simulink model "ALFlight3Wing"  (R2019a)
settings: Solver=VariableStepAuto  StartTime=0.0  StopTime=100  RelTol=1e-3
InitFcn:
  | Ts=.05
  | load('goodMPC.mat')
  | %load('fault2mpc.mat')
  | global counts
  | counts=0
  | 
  | An=[-0.0220400000000000,0.00142200000000000,0,-32.1700000000000,0,0,0,0,0,0;-0.0575900000000000,-0.394300000000000,871,0,0,0,0,0,0,0;-9.50000000000000e-05,-0.00179300000000000,-0.546800000000000,0,0,0,0,0,0,0;0,0,1,0,0,0,0,0,0,0;0,0,0,0,-0.0639900000000000,0,-1,0.0369100000000000,0,0;0,0,0,0,-2.11100000000000,-0.504800000000000,0.193000000000000,0,0,0;0,0,0,0,0.773200000000000,0.0108700000000000,-0.179400000000000,0,0,0;0,0,0,0,0,1,0,0,0,0;0,0,0,0,0,0,1,0,0,0;0,1,0,0,0,0,0,0,0,0]
  | Bn=[0,1.91000000000000e-05,0,0;-18.5800000000000,0,0,0;-1.20000000000000,0,0,0;0,0,0,0;0,0,0,0.00839000000000000;0,0,0.184800000000000,0.105600000000000;0,0,-0.00869900000000000,-0.459100000000000;0,0,0,0;0,0,0,0;0,0,0,0]
  | 
  | 
  |  set_param('ALFlight3Wing/ConstantA','Value','An')
  |  set_param('ALFlight3Wing/ConstantB','Value','Bn')
model workspace (MAT data in the model file):
  Uncertainty = Simulink.Signal
  Uncertainty.DataType = 'double'
  Uncertainty.Dimensions = -1
  Uncertainty.DimensionsMode = 'auto'
  Uncertainty.Complexity = 'auto'
  Uncertainty.SampleTime = -1
  Uncertainty.SamplingMode = 'auto'
  Uncertainty.InitialValue = '10000'
values from neighbouring files (symbols this model uses):
  Af2 = [-0.02204 -0.05759 -9.5e-05 0 0 0 0 0 0 0 0.001422 -0.3943 ... (100 elements, 10x10)]    [UpdatedWorkspace.mat]    (also in current2.mat; finalWorkspace.mat)
  Bf2 = [0 -18.58 -1.2 0 0 0 0 0 0 0 1.91e-05 0 ... (40 elements, 10x4)]    [UpdatedWorkspace.mat]    (also in current2.mat; finalWorkspace.mat)
  Cn = [1 0 0 0 0 0 0 0 0 0 0 0 ... (40 elements, 4x10)]    [UpdatedWorkspace.mat]    (also in current2.mat; finalWorkspace.mat)
  Dn = [0 0 0 0 0 0 0 0 0 0 0 0 ... (16 elements, 4x4)]    [UpdatedWorkspace.mat]    (also in current2.mat; finalWorkspace.mat)
  p = 15    [calcVar.m]    (also in chanceConstraintProgramming4.m = [norminv(.505),norminv(.6),norminv(.7),norminv(.8),norminv(.; dynamicsEst.m)
undefined symbols (not defined in the file or in its folder): Earth, iA, lastPcov, lastu, lastx, MDscale, mmpc_mvseq, mmpc_state, mmpc_ts, mmpc_u0, mmpc_xseq, mmpc_yseq, MVscale, nCC, nu, nud, nv, ny, nym, RMVscale, RYscale, ts, uoff, WGS84, xoff, Yscale
libraries: mpcsigdimcheck_private x44, simulink_extras x3, mpclib x2, commchan3 x1, aerolibtransform2 x1, aerolibfltsims x1, aerolibanimutils x1
(part 1 of 4)
settings Model: OrderedModelArguments=off  Creator=mschr  LastModifiedBy=mschr

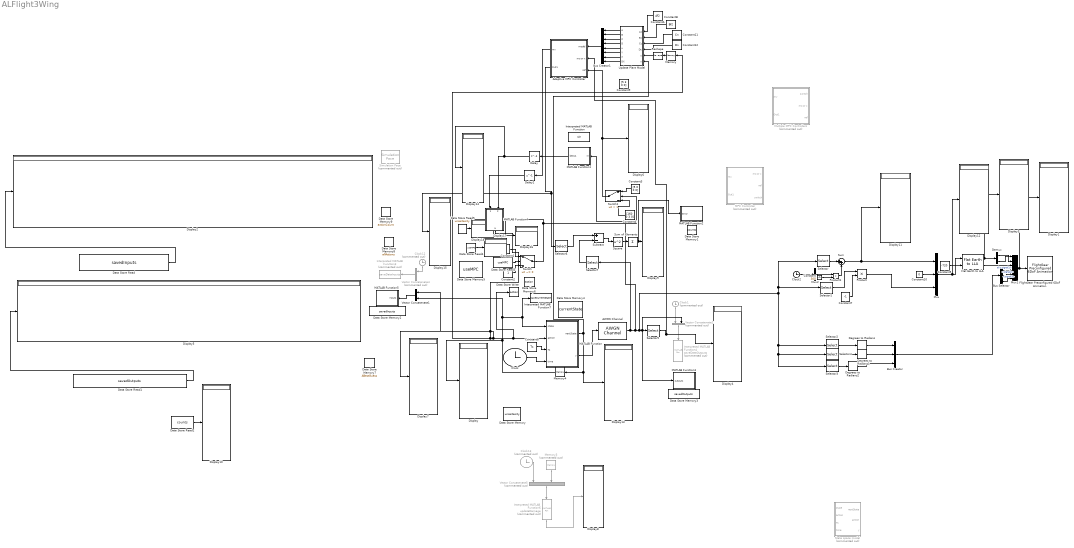
== system ALFlight3Wing ==
  AWGN Channel : commchan3/AWGN Channel  InputProcessing=Columns as channels (frame based)  seed=67  noiseMode="Signal to noise ratio  (SNR)"  EbNodB=50  EsNodB=10  SNRdB=100  bitsPerSym=1  Ps=1  Tsym=1  variance=1
      settings: SourceProductName=Communications Toolbox
  Adaptive MPC Controller : Subsystem  AncestorBlock=mpclib/Adaptive MPC Controller  SCDEnableBlockLinearizationSpecification=on  InitFcn=ampcblock_InitFcn  StartFcn=ampcblock_StartFcn  mask(Adaptive MPC){mpcobj=mpcNominalAdaptive, x0=, enable_value=0, updateMPCinCallerWorkspace=on, md_inport=off, mv_inport=off, uref_inport=off, return_cost=off, return_mvseq=off, return_qpstatus=off, return_xseq=off, return_state=off, return_ovseq=off, state_inport=off, isltv_plant=off, umin_inport=off, umax_inport=off, ymin_inport=off, ymax_inport=off, cc_inport=off, ywt_inport=off, uwt_inport=off, duwt_inport=off, rhoeps_inport=off, pm_inport=off, MaximumP=10, HorizonChoice=FixedHorizon, BlockDataType=double, SampleTimeInherited=off, switch_inport=off}
      mask prompts: mpcobj "MPC:general:BlgAMPC"; x0 "MPC:general:BlgState"; enable_value "Value enabling optimization"; updateMPCinCallerWorkspace "Update MPC object in caller workspace"; md_inport "MPC:general:BlgMD"; mv_inport "MPC:general:BlgEXTMV"; uref_inport "MPC:general:BlgMVTARGET"; return_cost "MPC:general:BlgCOST"; return_mvseq "MPC:general:BlgMVSEQ"; return_qpstatus "MPC:general:BlgQPSTATUS"; return_xseq "MPC:general:BlgXSEQ"; return_state "MPC:general:BlgESTSTATE"; return_ovseq "MPC:general:BlgOVSEQ"; state_inport "MPC:general:BlgXKK"; isltv_plant "MPC:general:BlgLTV"; umin_inport "MPC:general:BlgMVMin"; umax_inport "MPC:general:BlgMVMax"; ymin_inport "MPC:general:BlgOVMin"; ymax_inport "MPC:general:BlgOVMax"; cc_inport "Custom constraints (E, F, G, S)"; ywt_inport "MPC:general:BlgYWT"; uwt_inport "MPC:general:BlgUWT"; duwt_inport "MPC:general:BlgDUWT"; rhoeps_inport "MPC:general:BlgECRWT"; pm_inport "MPC:general:BlgPM"; MaximumP "MPC:general:BlgMaximumP"; HorizonChoice "Simulink:Variants:LabelComboBox"; BlockDataType "MPC:general:BlgDATATYPE"; SampleTimeInherited "MPC:general:BlgTS"; switch_inport "MPC:general:BlgSWITCH"
      mask help: MPC:utility:MaskDescAdaptiveMPC1
      mask init:
      | [blk,ts,A,B,C,D,isQP,strmoorx,nmoorx,nu,nv,ny,nx,nym,nud,...
      |     degrees,lastPcov,H,Hinv,Linv,iA,Ac,Kx,Ku1,Kut,Kr,Kv,...
      |     Mlim,Mx,Mu1,Mv,z_degrees,utarget,...
      |     lastx,lastu,p,xoff,uoff,yoff,voff,myoff,no_md,no_ref,...
      |     maxiter,CustomSolver,CustomSolverCodeGen,UseWarmStart,UseSuboptimalSolution,...
      |     nxQP,openloopflag,no_ym,no_mv,no_uref,...
      |     no_umin,no_umax,no_ymin,no_ymax,no_cc,...
      |     no_switch,CustomEstimation,...
      |     no_ywt, no_uwt, no_duwt, no_rhoeps,...
      |     Wy,Wdu,Jm,SuJm,Su1,Sx,Hv,Wu,I1,...
      |     isAdaptive, isLTV, Mrows, nCC, Ecc, Fcc, Scc, Gcc, Cid, Did, ...
      |     nxp, nup, nxid, mvindex, mdindex, unindex, myindex, ...
      |     Uscale, Yscale, MVscale, MDscale, ...
      |     RYscale,RMYscale,RMVscale,RMDscale,no_p,no_m,p0] = ampcblock_MaskInitFcnParameter();
      | ampcblock_MaskInitFcnResize(gcb,nv,nu,ny,nCC);
      mask Help: eval('mpcCSHelp(''MPCmaskAdaptive'',''HelpBrowser'')');
      mask Callback pm_inport: mpcblocks_callbackPM(gcb);
      mask TypeOptions HorizonChoice: MPC/optimizer/LabelModeActiveChoice
      mask DialogControl mpcobj Prompt: Adaptive MPC Controller
      mask DialogControl x0 Prompt: Initial Controller State
      mask DialogControl Container5 Prompt: MPC:general:BlgTab1
      mask DialogControl Container6 Prompt: MPC:general:BlgBox11
      mask DialogControl md_inport Prompt: Measured disturbance (md)
      mask DialogControl mv_inport Prompt: External manipulated variable (ext.mv)
      mask DialogControl uref_inport Prompt: Targets for manipulated variables (mv.target)
      mask DialogControl Container7 Prompt: MPC:general:BlgBox12
      mask DialogControl return_cost Prompt: Optimal cost (cost)
      mask DialogControl return_mvseq Prompt: Optimal control sequence (mv.seq)
      mask DialogControl return_qpstatus Prompt: Optimization status (qp.status)
      mask DialogControl return_xseq Prompt: Optimal state sequence (x.seq)
      mask DialogControl return_state Prompt: Estimated controller states (est.state)
      mask DialogControl return_ovseq Prompt: Optimal output sequence (y.seq)
      mask DialogControl Container16 Prompt: MPC:general:BlgBox13
      mask DialogControl state_inport Prompt: Use custom state estimation instead of using the built-in Kalman filter (x[k|k])
      mask DialogControl Container9 Prompt: MPC:general:BlgTab2
      mask DialogControl Container19 Prompt: MPC:general:BlgBox20
      mask DialogControl isltv_plant Prompt: Linear Time-Varying (LTV) plants (model expects 3-D signals)
      mask DialogControl Container10 Prompt: MPC:general:BlgBox21
      mask DialogControl umin_inport Prompt: Lower MV limits (umin)
      mask DialogControl umax_inport Prompt: Upper MV limits (umax)
      mask DialogControl ymin_inport Prompt: Lower OV limits (ymin)
      mask DialogControl ymax_inport Prompt: Upper OV limits (ymax)
      mask DialogControl Container11 Prompt: MPC:general:BlgBox22
      mask DialogControl ywt_inport Prompt: OV weights (y.wt)
      mask DialogControl uwt_inport Prompt: MV weights (u.wt)
      mask DialogControl duwt_inport Prompt: MVRate weights (du.wt)
      mask DialogControl rhoeps_inport Prompt: Slack variable weight (ecr.wt)
      mask DialogControl Container17 Prompt: Prediction and Control Horizons
      mask DialogControl pm_inport Prompt: Adjust prediction horizon (p) and control horizon (m) at run time
      mask DialogControl MaximumP Prompt: Maximum prediction horizon
      mask DialogControl HorizonChoice Prompt: Label mode active choice:
      mask DialogControl Container13 Prompt: MPC:general:BlgTab3
      mask DialogControl Container14 Prompt: MPC:general:BlgBox31
      mask DialogControl BlockDataType Prompt: Block Data Type
      mask DialogControl Container15 Prompt: MPC:general:BlgBox32
      mask DialogControl SampleTimeInherited Prompt: Inherit sample time (must be the same as controller sample time)
      mask DialogControl Container18 Prompt: MPC:general:BlgBox33
      mask DialogControl switch_inport Prompt: Use external signal to enable or disable optimization (switch)
      mask Display:
      | fprintf('Adaptive\nMPC');
      | port_label('output', 1, 'mv')
      | port_label('input', 1, 'model')
      | port_label('input', 2, 'mo')
      | port_label('input', 3, 'ref')
  Bus Creator : BusCreator  Inputs=3
  Bus Selector : BusSelector  OutputSignals=signal1,signal2,signal3
  Bus Creator1 : BusCreator  Inputs=8
  Clock : Clock
  Clock1 : Clock  Commented=on
  Clock12 : Clock  Commented=on
  Clock13 : Clock  Commented=on
  Clock2 : Clock
  Constant : Constant  Value=300  SampleTime=.05
  Constant1 : Constant  Value=2
  Constant10 : Constant  Value=0
  Constant11 : Constant  Value=Cn
  Constant12 : Constant  Value=Dn
  Constant2 : Constant
  Constant3 : Constant  Value=[5 0 0 0]
  Constant4 : Constant  Value=[160 0 3 0]
  Constant5 : Constant  Value=-720
  Constant7 : Constant  Value=-1
  Constant8 : Constant  Value=Ts
  Constant9 : Constant  Value=[5 3 0 0]
  ConstantA : Constant  Value=Af2
  ConstantB : Constant  Value=Bf2
  Data Store Memory : DataStoreMemory  DataStoreName=uncertainty  ReadBeforeWriteMsg=warning  WriteAfterWriteMsg=warning  WriteAfterReadMsg=warning  InitialValue=10000  ShowAdditionalParam=off  OutDataTypeStr=double
  Data Store Memory1 : DataStoreMemory  DataStoreName=counts  ReadBeforeWriteMsg=warning  WriteAfterWriteMsg=warning  WriteAfterReadMsg=warning  ShowAdditionalParam=off  OutDataTypeStr=double
  Data Store Memory2 : DataStoreMemory  DataStoreName=savedInputs  ReadBeforeWriteMsg=warning  WriteAfterWriteMsg=warning  WriteAfterReadMsg=warning  InitialValue=zeros(15,5000)  ShowAdditionalParam=off  OutDataTypeStr=double
  Data Store Memory3 : DataStoreMemory  DataStoreName=savedOutputs  ReadBeforeWriteMsg=warning  WriteAfterWriteMsg=warning  WriteAfterReadMsg=warning  InitialValue=zeros(11,5000)  ShowAdditionalParam=off  OutDataTypeStr=double
  Data Store Memory4 : DataStoreMemory  DataStoreName=currentState  ReadBeforeWriteMsg=warning  WriteAfterWriteMsg=warning  WriteAfterReadMsg=warning  InitialValue=zeros(11,1)  ShowAdditionalParam=off  OutDataTypeStr=double
  Data Store Memory5 : DataStoreMemory  DataStoreName=useMPC  ReadBeforeWriteMsg=warning  WriteAfterWriteMsg=warning  WriteAfterReadMsg=warning  InitialValue=false  ShowAdditionalParam=off  OutDataTypeStr=boolean
  Data Store Memory6 : DataStoreMemory  DataStoreName=action  ReadBeforeWriteMsg=warning  WriteAfterWriteMsg=warning  WriteAfterReadMsg=warning  InitialValue=[0 0 0 0]  ShowAdditionalParam=off  OutDataTypeStr=double
  Data Store Memory7 : DataStoreMemory  DataStoreName=ABestGuess  ReadBeforeWriteMsg=warning  WriteAfterWriteMsg=warning  WriteAfterReadMsg=warning  InitialValue=zeros(15,11)  ShowAdditionalParam=off  OutDataTypeStr=double
  Data Store Memory8 : DataStoreMemory  DataStoreName=allActions  ReadBeforeWriteMsg=warning  WriteAfterWriteMsg=warning  WriteAfterReadMsg=warning  InitialValue=zeros(8,1)  ShowAdditionalParam=off  OutDataTypeStr=double
  Data Store Memory9 : DataStoreMemory  DataStoreName=actionCount  ReadBeforeWriteMsg=warning  WriteAfterWriteMsg=warning  WriteAfterReadMsg=warning  InitialValue=2  ShowAdditionalParam=off  OutDataTypeStr=double
  Data Store Read : DataStoreRead  DataStoreName=savedInputs
  Data Store Read1 : DataStoreRead  DataStoreName=savedOutputs
  Data Store Read2 : DataStoreRead  DataStoreName=counts
  Data Store Read3 : DataStoreRead  DataStoreName=useMPC
  Data Store Read4 : DataStoreRead  DataStoreName=useMPC
  Data Store Read5 : DataStoreRead  DataStoreName=uncertainty
  Data Store Write : DataStoreWrite  DataStoreName=action
  Degrees to Radians : simulink_extras/Transformations/Degrees to Radians
  Degrees to Radians1 : simulink_extras/Transformations/Degrees to Radians
  Degrees to Radians2 : simulink_extras/Transformations/Degrees to Radians
  Delay : Delay  DelayLength=1  InitialCondition=0
  Delay2 : Delay  DelayLength=1  InitialCondition=0
  Demux : Demux  Outputs=2
  Display{,1..18} (19 alike) : Display
  Flat Earth to LLA : aerolibtransform2/Flat Earth to LLA  units=English  ptype=Earth (WGS84)  F=1/298.257223563  R=20925646.3255  LL0=[21.31835828 -157.9232806]  psi=0
  FlightGear Preconfigured 6DoF Animation : aerolibfltsims/FlightGear Preconfigured 6DoF Animation  xFlightGearVersion=v2018.2  DestinationIpAddress=127.0.0.1  DestinationPort=5502  SampleTime=.05  packetVersion=24
      settings: SourceProductName=Aerospace Blockset
  Interpreted MATLAB Function : MATLABFcn
  Interpreted MATLAB Function3 : MATLABFcn  Commented=on  MATLABFcn=saveDataInputs  OutputDimensions=0
  Interpreted MATLAB Function4 : MATLABFcn  Commented=on  MATLABFcn=saveDataOutputs  OutputDimensions=0
  Interpreted MATLAB Function6 : MATLABFcn  Commented=on  MATLABFcn=updateDamage  OutputDimensions=4
  Interpreted MATLAB Function7 : MATLABFcn  MATLABFcn=saveCurrentState  OutputDimensions=0
  MATLAB Function : MATLAB Function  TreatAsAtomicUnit=on  SystemSampleTime=.05
      settings: MinAlgLoopOccurrences=on
  MATLAB Function1 : MATLAB Function  TreatAsAtomicUnit=on
      settings: MinAlgLoopOccurrences=on
  MATLAB Function2 : MATLAB Function  TreatAsAtomicUnit=on
  MATLAB Function3 : MATLAB Function  TreatAsAtomicUnit=on
  MATLAB Function4 : MATLAB Function  TreatAsAtomicUnit=on  SystemSampleTime=.05
      settings: MinAlgLoopOccurrences=on
  MATLAB Function5 : MATLAB Function  TreatAsAtomicUnit=on
  MPC Controller : Subsystem  Commented=on  AncestorBlock=mpclib/MPC Controller  SCDEnableBlockLinearizationSpecification=on  InitFcn=impcblock_InitFcn  StartFcn=impcblock_StartFcn  mask(MPC){mpcobj=mpc1, x0=, is_multiple=0, enable_value=0, return_u0=off, updateMPCinCallerWorkspace=on, md_inport=off, mv_inport=off, uref_inport=off, return_cost=off, return_mvseq=off, return_qpstatus=off, return_xseq=off, return_state=off, return_ovseq=off, state_inport=off, umin_inport=off, umax_inport=off, ymin_inport=off, ymax_inport=off, cc_inport=off, ywt_inport=off, uwt_inport=off, duwt_inport=off, rhoeps_inport=off, pm_inport=off, MaximumP=10, HorizonChoice=FixedHorizon, n_ts=0.05, n_p=70, n_mv=4, n_md=0, n_ud=0, n_mo=4, n_uo=0, BlockDataType=double, SampleTimeInherited=off, switch_inport=on}
      mask prompts: mpcobj "MPC:general:BlgIMPC"; x0 "MPC:general:BlgState"; is_multiple "Flag indicating the block is part of multiple blocks"; enable_value "Value enabling optimization"; return_u0 "Export u0"; updateMPCinCallerWorkspace "Update MPC object in the caller workspace"; md_inport "MPC:general:BlgMD"; mv_inport "MPC:general:BlgEXTMV"; uref_inport "MPC:general:BlgMVTARGET"; return_cost "MPC:general:BlgCOST"; return_mvseq "MPC:general:BlgMVSEQ"; return_qpstatus "MPC:general:BlgQPSTATUS"; return_xseq "MPC:general:BlgXSEQ"; return_state "MPC:general:BlgESTSTATE"; return_ovseq "MPC:general:BlgOVSEQ"; state_inport "MPC:general:BlgXKK"; umin_inport "MPC:general:BlgMVMin"; umax_inport "MPC:general:BlgMVMax"; ymin_inport "MPC:general:BlgOVMin"; ymax_inport "MPC:general:BlgOVMax"; cc_inport "Custom constraints (E, F, G, S)"; ywt_inport "MPC:general:BlgYWT"; uwt_inport "MPC:general:BlgUWT"; duwt_inport "MPC:general:BlgDUWT"; rhoeps_inport "MPC:general:BlgECRWT"; pm_inport "MPC:general:BlgPM"; MaximumP "MPC:general:BlgMaximumP"; HorizonChoice "Simulink:Variants:LabelComboBox"; n_ts "MPC:general:BlgSampleTime"; n_p "MPC:general:BlgNumP"; n_mv "MPC:general:BlgNumMV"; n_md "MPC:general:BlgNumMD"; n_ud "MPC:general:BlgNumUD"; n_mo "MPC:general:BlgNumMO"; n_uo "MPC:general:BlgNumUO"; BlockDataType "MPC:general:BlgDATATYPE"; SampleTimeInherited "MPC:general:BlgTS"; switch_inport "MPC:general:BlgSWITCH"
      mask help: MPC:utility:MaskDescMPC1
      mask init:
      | [blk,ts,A,Cm,Bu,Bv,Dvm,isQP,strmoorx,nmoorx,nu,nv,ny,nx,nym...
      |     degrees,L,M,H,Hinv,Linv,iA,Ac,Kx,Ku1,Kut,Kr,Kv,...
      |     Mlim,Mx,Mu1,Mv,z_degrees,utarget,...
      |     lastx,lastu,p,xoff,uoff,yoff,voff,myoff,no_md,no_ref,...
      |     maxiter,CustomSolver,CustomSolverCodeGen,UseWarmStart,UseSuboptimalSolution,...
      |     nxQP,openloopflag,no_ym,no_mv,no_uref,...
      |     no_umin,no_umax,no_ymin,no_ymax,no_cc,...
      |     no_switch,CustomEstimation,...
      |     no_ywt, no_uwt, no_duwt, no_rhoeps,...
      |     Wy,Wdu,Jm,SuJm,Su1,Sx,Hv,Wu,I1,...
      |     isAdaptive, C, Dv, Mrows, nCC, Ecc, Fcc, Scc, Gcc, ...
      |     nxp, nxindist, mvindex, mdindex, unindex, myindex, ...
      |     Uscale, Yscale, MVscale, MDscale, ...
      |     RYscale,RMYscale,RMVscale,RMDscale,no_p,no_m,p0] = impcblock_MaskInitFcnParameter(return_cost,return_mvseq,return_xseq,return_ovseq);
      | impcblock_MaskInitFcnResize(gcb,nv,nu,ny,nCC);
      mask Help: eval('mpcCSHelp(''MPCmask'',''HelpBrowser'')');
      mask Callback md_inport: impcblock_mdcallback(gcb);
      mask Callback pm_inport: mpcblocks_callbackPM(gcb);
      mask TypeOptions HorizonChoice: MPC/optimizer/LabelModeActiveChoice
      mask DialogControl mpcobj Prompt: MPC Controller
      mask DialogControl design_button Prompt: MPC:general:BlgDesignButton
      mask DialogControl design_button Callback: mpc_designcallback(gcbh)
      mask DialogControl x0 Prompt: Initial Controller State
      mask DialogControl review_button Prompt: MPC:general:BlgReviewButton
      mask DialogControl review_button Callback: mpc_reviewcallback(gcbh)
      mask DialogControl OptionGroup Prompt: MPC:general:BlgBlockOptions
      mask DialogControl GeneralTab Prompt: MPC:general:BlgTab1
      mask DialogControl Container6 Prompt: MPC:general:BlgBox11
      mask DialogControl md_inport Prompt: Measured disturbance (md)
      mask DialogControl mv_inport Prompt: External manipulated variable (ext.mv)
      mask DialogControl uref_inport Prompt: Targets for manipulated variables (mv.target)
      mask DialogControl Container7 Prompt: MPC:general:BlgBox12
      mask DialogControl return_cost Prompt: Optimal cost (cost)
      mask DialogControl return_mvseq Prompt: Optimal control sequence (mv.seq)
      mask DialogControl return_qpstatus Prompt: Optimization status (qp.status)
      mask DialogControl return_xseq Prompt: Optimal state sequence (x.seq)
      mask DialogControl return_state Prompt: Estimated controller states (est.state)
      mask DialogControl return_ovseq Prompt: Optimal output sequence (y.seq)
      mask DialogControl Container14 Prompt: MPC:general:BlgBox13
      mask DialogControl state_inport Prompt: Use custom state estimation instead of using the built-in Kalman filter (x[k|k])
      mask DialogControl OnlineTab Prompt: MPC:general:BlgTab2
      mask DialogControl Container6_copy Prompt: MPC:general:BlgBox21
      mask DialogControl umin_inport Prompt: Lower MV limits (umin)
      mask DialogControl umax_inport Prompt: Upper MV limits (umax)
      mask DialogControl ymin_inport Prompt: Lower OV limits (ymin)
      mask DialogControl ymax_inport Prompt: Upper OV limits (ymax)
      mask DialogControl Container7_copy Prompt: MPC:general:BlgBox22
      mask DialogControl ywt_inport Prompt: OV weights (y.wt)
      mask DialogControl uwt_inport Prompt: MV weights (u.wt)
      mask DialogControl duwt_inport Prompt: MVRate weights (du.wt)
      mask DialogControl rhoeps_inport Prompt: Slack variable weight (ecr.wt)
      mask DialogControl Container16 Prompt: MPC:general:BlgBox23
      mask DialogControl pm_inport Prompt: Adjust prediction horizon (p) and control horizon (m) at run time
      mask DialogControl MaximumP Prompt: Maximum prediction horizon
      mask DialogControl HorizonChoice Prompt: Label mode active choice:
      mask DialogControl SignalSizeTab Prompt: MPC:general:BlgDefaultConditions
      mask DialogControl Container24 Prompt: MPC:general:BlgDefaultSampleTime
      mask DialogControl n_ts Prompt: Sample time
      mask DialogControl n_p Prompt: Prediction Horizon
      mask DialogControl InputSizeGroup Prompt: MPC:general:BlgDefaultInputSize
      mask DialogControl n_mv Prompt: Number of manipulated variables
      mask DialogControl n_md Prompt: Number of measured disturbances
      mask DialogControl n_ud Prompt: Number of unmeasured disturbances
      mask DialogControl OutputSizeGroup Prompt: MPC:general:BlgDefaultOutputSize
      mask DialogControl n_mo Prompt: Number of measured outputs
      mask DialogControl n_uo Prompt: Number of unmeasured outputs
      mask DialogControl OtherTab Prompt: MPC:general:BlgTab3
      mask DialogControl Container6_copy_copy Prompt: MPC:general:BlgBox31
      mask DialogControl BlockDataType Prompt: Block Data Type
      mask DialogControl Container7_copy_copy Prompt: MPC:general:BlgBox32
      mask DialogControl SampleTimeInherited Prompt: Inherit sample time (must be the same as controller sample time)
      mask DialogControl Container17 Prompt: MPC:general:BlgBox33
      mask DialogControl switch_inport Prompt: Use external signal to enable or disable optimization (switch)
      mask Display:
      | fprintf('MPC');
      | port_label('output', 1, 'mv')
      | port_label('input', 1, 'mo')
      | port_label('input', 2, 'ref')
      | port_label('input', 3, 'switch')
  Memory : Memory  InitialCondition=zeros(4,1)
  Memory3 : Memory  Commented=on  InitialCondition=zeros(11,1)  InheritSampleTime=on
  Memory4 : Memory  InitialCondition=zeros(11,1)  InheritSampleTime=on  LinearizeAsDelay=on
  Multiple MPC Controllers : Subsystem  Commented=on  AncestorBlock=mpclib/Multiple MPC Controllers  StartFcn=mmpcblock_StartFcn  mask(Multiple MPC){mpcobjs={'mpc1','fault1MPC'}, x0s={'[]','[]'}, Nmpc=1, theMPC=1, nmv=1, nmo=1, nmd=1, nts=1, md_inport_multiple=off, mv_inport_multiple=off, uref_inport_multiple=off, return_cost_multiple=off, return_mvseq_multiple=off, return_qpstatus_multiple=off, return_xseq_multiple=off, return_state_multiple=off, return_ovseq_multiple=off, state_inport_multiple=off, umin_inport_multiple=off, umax_inport_multiple=off, ymin_inport_multiple=off, ymax_inport_multiple=off, ywt_inport_multiple=off, uwt_inport_multiple=off, duwt_inport_multiple=off, rhoeps_inport_multiple=off, BlockDataType_multiple=double, SampleTimeInherited_multiple=off}
      mask prompts: mpcobjs "MPC:general:BlgMMPC"; x0s "MPC:general:BlgStates"; Nmpc "Number of multiple MPC controllers"; theMPC "Currently selected MPC controller"; nmv "Number of MVs"; nmo "Number of MOa"; nmd "Number of MDs"; nts "Sample Time"; md_inport_multiple "MPC:general:BlgMD"; mv_inport_multiple "MPC:general:BlgEXTMV"; uref_inport_multiple "MPC:general:BlgMVTARGET"; return_cost_multiple "MPC:general:BlgCOST"; return_mvseq_multiple "MPC:general:BlgMVSEQ"; return_qpstatus_multiple "MPC:general:BlgQPSTATUS"; return_xseq_multiple "MPC:general:BlgXSEQ"; return_state_multiple "MPC:general:BlgESTSTATE"; return_ovseq_multiple "MPC:general:BlgOVSEQ"; state_inport_multiple "MPC:general:BlgXKK"; umin_inport_multiple "MPC:general:BlgMVMin"; umax_inport_multiple "MPC:general:BlgMVMax"; ymin_inport_multiple "MPC:general:BlgOVMin"; ymax_inport_multiple "MPC:general:BlgOVMax"; ywt_inport_multiple "MPC:general:BlgYWT"; uwt_inport_multiple "MPC:general:BlgUWT"; duwt_inport_multiple "MPC:general:BlgDUWT"; rhoeps_inport_multiple "MPC:general:BlgECRWT"; BlockDataType_multiple "MPC:general:BlgDATATYPE"; SampleTimeInherited_multiple "MPC:general:BlgTS"
      mask help: MPC:utility:MaskDescMultipleMPC1
      mask init:
      | [mmpc_u0, mmpc_mvseq, mmpc_xseq, mmpc_yseq, mmpc_state, mmpc_ts] = mmpcblock_MaskInitFcnResize(gcb);
      mask Help: eval('mpcCSHelp(''MPCmaskMultiple'',''HelpBrowser'')');
      mask DialogControl mpcobjs Prompt: Cell Array of MPC Controllers
      mask DialogControl x0s Prompt: Cell Array of Initial Controller States
      mask DialogControl Container3 Prompt: MPC:general:BlgBlockOptions
      mask DialogControl Container5 Prompt: MPC:general:BlgTab1
      mask DialogControl Container6 Prompt: MPC:general:BlgBox11
      mask DialogControl md_inport_multiple Prompt: Measured disturbance (md)
      mask DialogControl mv_inport_multiple Prompt: External manipulated variable (ext.mv)
      mask DialogControl uref_inport_multiple Prompt: Targets for manipulated variables (mv.target)
      mask DialogControl Container6_copy Prompt: MPC:general:BlgBox12
      mask DialogControl return_cost_multiple Prompt: Optimal cost (cost)
      mask DialogControl return_mvseq_multiple Prompt: Optimal control sequence (mv.seq)
      mask DialogControl return_qpstatus_multiple Prompt: Optimization status (qp.status)
      mask DialogControl return_xseq_multiple Prompt: Optimal state sequence (x.seq)
      mask DialogControl return_state_multiple Prompt: Estimated controller states (est.state)
      mask DialogControl return_ovseq_multiple Prompt: Optimal output sequence (y.seq)
      mask DialogControl Container16 Prompt: MPC:general:BlgBox13
      mask DialogControl state_inport_multiple Prompt: Use custom state estimation instead of using the built-in Kalman filter (x[k|k])
      mask DialogControl Container10 Prompt: MPC:general:BlgTab2
      mask DialogControl Container6_copy_copy Prompt: MPC:general:BlgBox21
      mask DialogControl umin_inport_multiple Prompt: Lower MV limits (umin)
      mask DialogControl umax_inport_multiple Prompt: Upper MV limits (umax)
      mask DialogControl ymin_inport_multiple Prompt: Lower OV limits (ymin)
      mask DialogControl ymax_inport_multiple Prompt: Upper OV limits (ymax)
      mask DialogControl Container14 Prompt: MPC:general:BlgBox22
      mask DialogControl ywt_inport_multiple Prompt: OV weights (y.wt)
      mask DialogControl uwt_inport_multiple Prompt: MV weights (u.wt)
      mask DialogControl duwt_inport_multiple Prompt: MVRate weights (du.wt)
      mask DialogControl rhoeps_inport_multiple Prompt: Slack variable weight (ecr.wt)
      mask DialogControl Container10_copy Prompt: MPC:general:BlgTab3
      mask DialogControl Container6_copy_copy_copy Prompt: MPC:general:BlgBox31
      mask DialogControl BlockDataType_multiple Prompt: Block Data Type
      mask DialogControl Container6_copy_copy_copy_copy Prompt: MPC:general:BlgBox32
      mask DialogControl SampleTimeInherited_multiple Prompt: Inherit sample time (must be the same as controller sample time)
      mask Display:
      | fprintf('Multiple\nMPC');
      | port_label('output', 1, 'mv')
      | port_label('input', 1, 'switch')
      | port_label('input', 2, 'mo')
      | port_label('input', 3, 'ref')
  Mux : Mux  Inputs=3
  Mux1 : Mux  Inputs=6
  Mux2 : Mux  Inputs=1
  Product : Product
  Product1 : Product
  Reshape : Reshape  OutputDimensionality=Customize  OutputDimensions=[4,1]
  Selector : Selector  InputPortWidth=11  IndexOptions=Index vector (dialog)  Indices=10  OutputSizes=1
  Selector1 : Selector  InputPortWidth=11  IndexOptions=Index vector (dialog)  Indices=11  OutputSizes=1
  Selector2 : Selector  InputPortWidth=11  IndexOptions=Index vector (dialog)  Indices=8  OutputSizes=1
  Selector3 : Selector  InputPortWidth=11  IndexOptions=Index vector (dialog)  Indices=9  OutputSizes=1
  Selector4 : Selector  InputPortWidth=11  IndexOptions=Index vector (dialog)  Indices=4  OutputSizes=1
  Selector5 : Selector  InputPortWidth=11  IndexOptions=Index vector (dialog)  Indices=[1 8 9 11]  OutputSizes=1
  Selector6 : Selector  InputPortWidth=12  IndexOptions=Index vector (dialog)  Indices=[1 2 3 4 5 6 7 8 9]  OutputSizes=1
  Selector7 : Selector  InputPortWidth=11  IndexOptions=Index vector (dialog)  Indices=[1 2 3 4 5 6 7 8 9]  OutputSizes=1
  Simulation Pace : aerolibanimutils/Simulation Pace  Commented=on  SimulationPace=10  SleepMode=Auto  OutputPaceError=off  SampleTime=1/30
  Square : Math  Operator=square  SaturateOnIntegerOverflow=on
  State space model : MATLAB Function  Commented=on  TreatAsAtomicUnit=on  SystemSampleTime=.05
      settings: MinAlgLoopOccurrences=on
  Subtract : Sum  Inputs=+-
  Sum : Sum  Inputs=|++
  Sum of Elements : Sum  Inputs=+
  Switch : Switch  Criteria=u2 ~= 0  Threshold=.01
  Switch1 : Switch  Criteria=u2 > Threshold  Threshold=1
  Update Plant Model : MATLAB Function  TreatAsAtomicUnit=on
  Vector Concatenate1 : Concatenate
  Vector Concatenate2 : Concatenate  Commented=on
  Vector Concatenate4 : Concatenate  Commented=on  NumInputs=3
  Vector Concatenate5 : Concatenate  Commented=on  NumInputs=4
  wires:
  Vector Concatenate2/1 -> Interpreted MATLAB Function4/1
  Clock1/1 -> Vector Concatenate2/1
  Constant8/1 -> MATLAB Function/3(Ts)
  Clock/1 -> MATLAB Function/4(time)
  Memory4/1 -> Vector Concatenate1/2, Interpreted MATLAB Function7/1, MATLAB Function/1(state), Display/1
  Constant3/1 -> Switch1/1
  Degrees to Radians2/1 -> Bus Creator/3
  Bus Selector/3 -> Mux1/6  "<signal3>"
  Degrees to Radians/1 -> Bus Creator/1
  Bus Selector/2 -> Mux1/5  "<signal2>"
  Degrees to Radians1/1 -> Bus Creator/2
  Selector2/1 -> Degrees to Radians/1
  Flat Earth to LLA/2 -> Mux1/3  "alt"
  Mux1/1 -> Display1/1, FlightGear Preconfigured 6DoF Animation/1
  Demux/1 -> Mux1/2
  Constant7/1 -> Product/2
  Constant10/1 -> Mux/2
  Selector3/1 -> Degrees to Radians2/1
  Flat Earth to LLA/1 -> Display3/1, Demux/1
  Bus Selector/1 -> Mux1/4  "<signal1>"
  Sum/1 -> Display11/1, Mux/1
  Mux/1 -> Flat Earth to LLA/1, Display12/1
  Selector4/1 -> Degrees to Radians1/1
  Bus Creator/1 -> Bus Selector/1
  Product/1 -> Mux/3
  Selector1/1 -> Product/1
  Constant5/1 -> Flat Earth to LLA/2
  Demux/2 -> Mux1/1
  MATLAB Function4/1(a) -> Vector Concatenate1/1, Memory/1, MATLAB Function/2(action), Data Store Write/1, Display7/1
  Vector Concatenate4/1 -> Interpreted MATLAB Function3/1
  Clock12/1 -> Vector Concatenate4/1
  Vector Concatenate5/1 -> Interpreted MATLAB Function6/1
  Memory3/1 -> Vector Concatenate5/3
  Clock13/1 -> Vector Concatenate5/1
  Interpreted MATLAB Function6/1 -> Display8/1
  Selector/1 -> Sum/1
  MATLAB Function1/1(bestA) -> Delay/1
  Constant/1 -> Product1/2
  Product1/1 -> Sum/2
  Mux2/1 -> Product1/1
  Clock2/1 -> Mux2/1
  Selector6/1 -> Subtract/1
  Subtract/1 -> Square/1
  Square/1 -> Sum of Elements/1
  Sum of Elements/1 -> MATLAB Function2/1(error), Display9/1
  Vector Concatenate1/1 -> MATLAB Function5/1(inputs)
  MATLAB Function/2(y) -> AWGN Channel/1
  Adaptive MPC Controller/1(mv) -> Delay2/1
  Data Store Read/1 -> Display2/1
  Data Store Read1/1 -> Display5/1
  Data Store Read2/1 -> Display10/1
  Delay/1 -> Display14/1, MATLAB Function4/2(actionAL)
  Delay2/1 -> MATLAB Function4/1(actionMPC)
  Selector7/1 -> Subtract/2
  Adaptive MPC Controller/2(Out1) -> Selector6/1, Display15/1
  AWGN Channel/1 -> Selector7/1, MATLAB Function1/1(in), Selector1/1, Selector/1, Selector2/1, Selector4/1, Selector3/1, Vector Concatenate2/2, MATLAB Function3/1(outputs), Selector5/1
  Data Store Read3/1 -> Switch/2
  Constant1/1 -> Switch/1
  Constant2/1 -> Switch/3
  Switch/1 -> Display16/1, Switch1/2
  Data Store Read4/1 -> Display17/1
  Data Store Read5/1 -> Display18/1
  Constant4/1 -> Switch1/3
  Switch1/1 -> Adaptive MPC Controller/3(ref), Display6/1
  Memory/1 -> Reshape/1
  MATLAB Function/1(nextState) -> Display13/1, Memory4/1, Update Plant Model/6(x)
  Update Plant Model/7(X) -> Bus Creator1/7
  Update Plant Model/8(DX) -> Bus Creator1/8
  Update Plant Model/6(Y) -> Bus Creator1/6
  Update Plant Model/3(C) -> Bus Creator1/3
  Update Plant Model/1(A) -> Bus Creator1/1
  Update Plant Model/4(D) -> Bus Creator1/4
  Update Plant Model/2(B) -> Bus Creator1/2
  Reshape/1 -> Update Plant Model/5("u ")
  Constant12/1 -> Update Plant Model/4(Dc)
  ConstantB/1 -> Update Plant Model/2(Bc)
  Constant11/1 -> Update Plant Model/3(Cc)
  ConstantA/1 -> Update Plant Model/1(Ac)
  Selector5/1 -> Adaptive MPC Controller/2(mo or x), Display4/1
  Bus Creator1/1 -> Adaptive MPC Controller/1(model)
  Update Plant Model/5(u) -> Bus Creator1/5

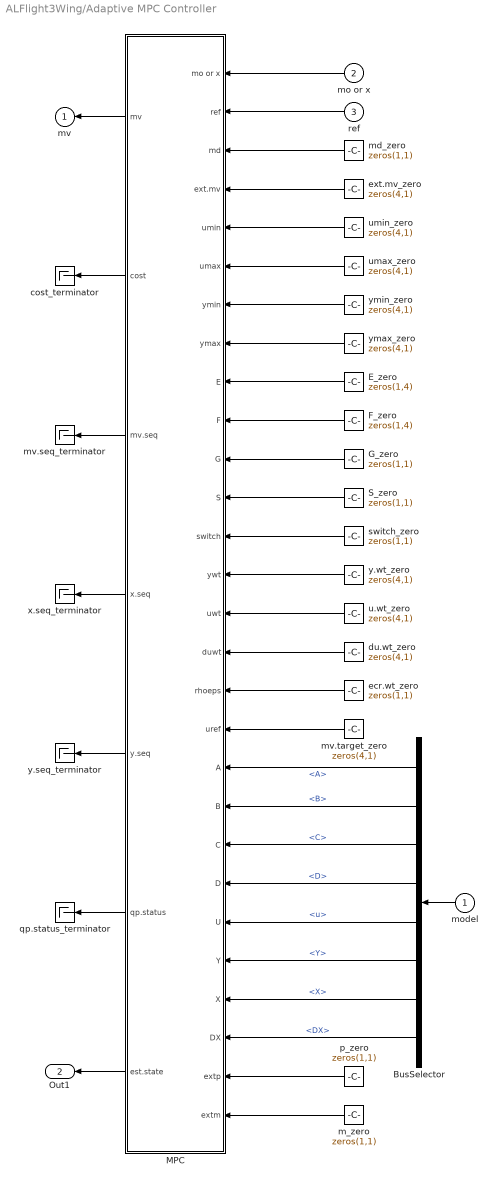
== system ALFlight3Wing/Adaptive MPC Controller ==
  model : Inport
  mo or x : Inport  Port=2
  ref : Inport  Port=3
  BusSelector : BusSelector  OutputSignals=A,B,C,D,u,Y,X,DX
  E_zero : Constant  Value=zeros(1,4)  VectorParams1D=off  OutDataTypeStr=BlockDataType
  F_zero : Constant  Value=zeros(1,4)  VectorParams1D=off  OutDataTypeStr=BlockDataType
  G_zero : Constant  Value=zeros(1,1)  VectorParams1D=off  OutDataTypeStr=BlockDataType
  MPC : Subsystem
  S_zero : Constant  Value=zeros(1,1)  VectorParams1D=off  OutDataTypeStr=BlockDataType
  cost_terminator : Terminator
  du.wt_zero : Constant  Value=zeros(4,1)  OutDataTypeStr=BlockDataType
  ecr.wt_zero : Constant  Value=zeros(1,1)  OutDataTypeStr=BlockDataType
  ext.mv_zero : Constant  Value=zeros(4,1)  OutDataTypeStr=BlockDataType
  m_zero : Constant  Value=zeros(1,1)  OutDataTypeStr=BlockDataType
  md_zero : Constant  Value=zeros(1,1)  OutDataTypeStr=BlockDataType
  mv.seq_terminator : Terminator
  mv.target_zero : Constant  Value=zeros(4,1)  OutDataTypeStr=BlockDataType
  p_zero : Constant  Value=zeros(1,1)  OutDataTypeStr=BlockDataType
  qp.status_terminator : Terminator
  switch_zero : Constant  Value=zeros(1,1)  OutDataTypeStr=BlockDataType
  u.wt_zero : Constant  Value=zeros(4,1)  OutDataTypeStr=BlockDataType
  umax_zero : Constant  Value=zeros(4,1)  OutDataTypeStr=BlockDataType
  umin_zero : Constant  Value=zeros(4,1)  OutDataTypeStr=BlockDataType
  x.seq_terminator : Terminator
  y.seq_terminator : Terminator
  y.wt_zero : Constant  Value=zeros(4,1)  OutDataTypeStr=BlockDataType
  ymax_zero : Constant  Value=zeros(4,1)  OutDataTypeStr=BlockDataType
  ymin_zero : Constant  Value=zeros(4,1)  OutDataTypeStr=BlockDataType
  mv : Outport
  Out1 : Outport  Port=2
  wires:
  m_zero/1 -> MPC/28(extm)
  p_zero/1 -> MPC/27(extp)
  MPC/5(y.seq) -> y.seq_terminator/1
  MPC/4(x.seq) -> x.seq_terminator/1
  G_zero/1 -> MPC/11(G)
  F_zero/1 -> MPC/10(F)
  E_zero/1 -> MPC/9(E)
  S_zero/1 -> MPC/12(S)
  MPC/7(est.state) -> Out1/1
  y.wt_zero/1 -> MPC/14(ywt)
  switch_zero/1 -> MPC/13(switch)
  ymin_zero/1 -> MPC/7(ymin)
  umax_zero/1 -> MPC/6(umax)
  umin_zero/1 -> MPC/5(umin)
  u.wt_zero/1 -> MPC/15(uwt)
  ymax_zero/1 -> MPC/8(ymax)
  du.wt_zero/1 -> MPC/16(duwt)
  ecr.wt_zero/1 -> MPC/17(rhoeps)
  mv.target_zero/1 -> MPC/18(uref)
  ext.mv_zero/1 -> MPC/4(ext.mv)
  BusSelector/8 -> MPC/26(DX)  "<DX>"
  BusSelector/7 -> MPC/25(X)  "<X>"
  BusSelector/6 -> MPC/24(Y)  "<Y>"
  BusSelector/5 -> MPC/23(U)  "<u>"
  model/1 -> BusSelector/1
  BusSelector/4 -> MPC/22(D)  "<D>"
  BusSelector/3 -> MPC/21(C)  "<C>"
  BusSelector/2 -> MPC/20(B)  "<B>"
  BusSelector/1 -> MPC/19(A)  "<A>"
  MPC/6(qp.status) -> qp.status_terminator/1
  MPC/3(mv.seq) -> mv.seq_terminator/1
  MPC/2(cost) -> cost_terminator/1
  ref/1 -> MPC/2(ref)
  mo or x/1 -> MPC/1(mo or x)
  MPC/1(mv) -> mv/1
  md_zero/1 -> MPC/3(md)

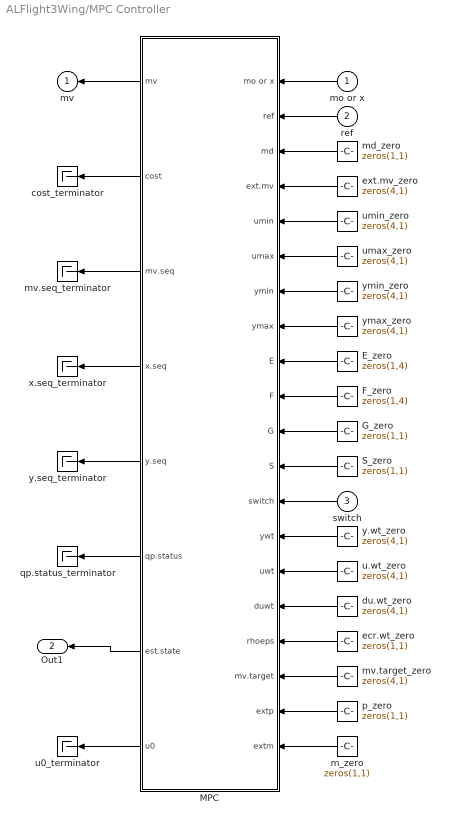
== system ALFlight3Wing/MPC Controller ==
  mo or x : Inport
  ref : Inport  Port=2
  switch : Inport  Port=3
  E_zero : Constant  Value=zeros(1,4)  VectorParams1D=off  OutDataTypeStr=BlockDataType
  F_zero : Constant  Value=zeros(1,4)  VectorParams1D=off  OutDataTypeStr=BlockDataType
  G_zero : Constant  Value=zeros(1,1)  VectorParams1D=off  OutDataTypeStr=BlockDataType
  MPC : Subsystem
  S_zero : Constant  Value=zeros(1,1)  VectorParams1D=off  OutDataTypeStr=BlockDataType
  cost_terminator : Terminator
  du.wt_zero : Constant  Value=zeros(4,1)  OutDataTypeStr=BlockDataType
  ecr.wt_zero : Constant  Value=zeros(1,1)  OutDataTypeStr=BlockDataType
  ext.mv_zero : Constant  Value=zeros(4,1)  OutDataTypeStr=BlockDataType
  m_zero : Constant  Value=zeros(1,1)  OutDataTypeStr=BlockDataType
  md_zero : Constant  Value=zeros(1,1)  OutDataTypeStr=BlockDataType
  mv.seq_terminator : Terminator
  mv.target_zero : Constant  Value=zeros(4,1)  OutDataTypeStr=BlockDataType
  p_zero : Constant  Value=zeros(1,1)  OutDataTypeStr=BlockDataType
  qp.status_terminator : Terminator
  u.wt_zero : Constant  Value=zeros(4,1)  OutDataTypeStr=BlockDataType
  u0_terminator : Terminator
  umax_zero : Constant  Value=zeros(4,1)  OutDataTypeStr=BlockDataType
  umin_zero : Constant  Value=zeros(4,1)  OutDataTypeStr=BlockDataType
  x.seq_terminator : Terminator
  y.seq_terminator : Terminator
  y.wt_zero : Constant  Value=zeros(4,1)  OutDataTypeStr=BlockDataType
  ymax_zero : Constant  Value=zeros(4,1)  OutDataTypeStr=BlockDataType
  ymin_zero : Constant  Value=zeros(4,1)  OutDataTypeStr=BlockDataType
  mv : Outport
  Out1 : Outport  Port=2
  wires:
  m_zero/1 -> MPC/20(extm)
  p_zero/1 -> MPC/19(extp)
  MPC/7(est.state) -> Out1/1
  MPC/6(qp.status) -> qp.status_terminator/1
  MPC/5(y.seq) -> y.seq_terminator/1
  MPC/4(x.seq) -> x.seq_terminator/1
  MPC/3(mv.seq) -> mv.seq_terminator/1
  MPC/2(cost) -> cost_terminator/1
  ext.mv_zero/1 -> MPC/4(ext.mv)
  mv.target_zero/1 -> MPC/18(mv.target)
  y.wt_zero/1 -> MPC/14(ywt)
  S_zero/1 -> MPC/12(S)
  G_zero/1 -> MPC/11(G)
  F_zero/1 -> MPC/10(F)
  E_zero/1 -> MPC/9(E)
  MPC/8(u0) -> u0_terminator/1
  ymax_zero/1 -> MPC/8(ymax)
  ymin_zero/1 -> MPC/7(ymin)
  umax_zero/1 -> MPC/6(umax)
  umin_zero/1 -> MPC/5(umin)
  u.wt_zero/1 -> MPC/15(uwt)
  ecr.wt_zero/1 -> MPC/17(rhoeps)
  du.wt_zero/1 -> MPC/16(duwt)
  MPC/1(mv) -> mv/1
  mo or x/1 -> MPC/1(mo or x)
  ref/1 -> MPC/2(ref)
  md_zero/1 -> MPC/3(md)
  switch/1 -> MPC/13(switch)

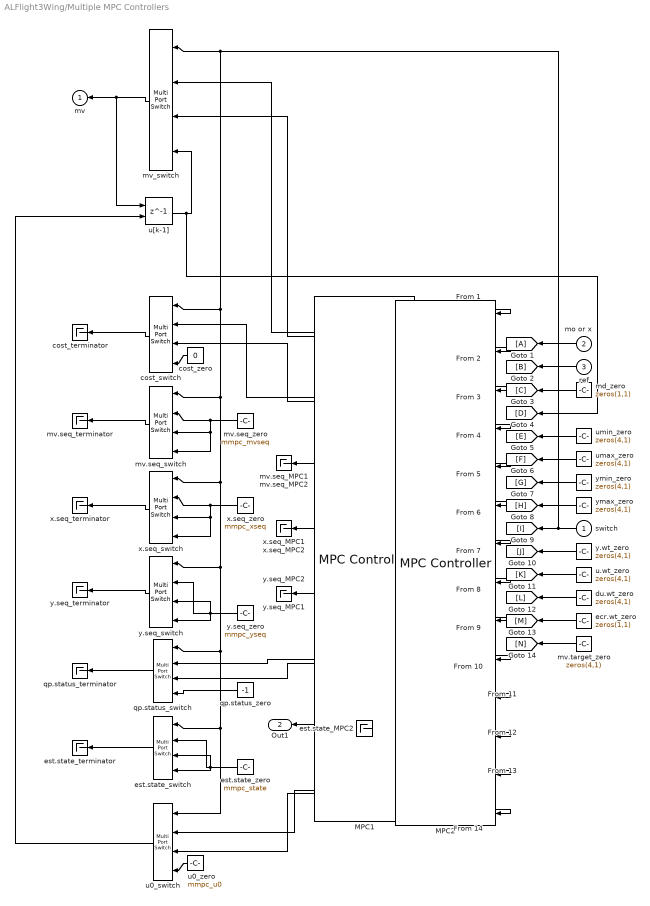
== system ALFlight3Wing/Multiple MPC Controllers ==
  switch : Inport
  mo or x : Inport  Port=2
  ref : Inport  Port=3
  MPC1 : mpclib/MPC Controller  SCDEnableBlockLinearizationSpecification=on  mpcobj=mpc1  x0=[]  is_multiple=1  enable_value=1  return_u0=on  updateMPCinCallerWorkspace=on  md_inport=on  mv_inport=on  uref_inport=on  return_cost=on  return_mvseq=on  return_qpstatus=on  return_xseq=on  return_state=on  return_ovseq=on  state_inport=off  umin_inport=on  umax_inport=on  ymin_inport=on  ymax_inport=on  cc_inport=off  ywt_inport=on  uwt_inport=on  duwt_inport=on  rhoeps_inport=on  pm_inport=off  MaximumP=10  HorizonChoice=FixedHorizon  n_ts=0.05  n_p=70  n_mv=4  n_md=0  n_ud=0  n_mo=4  n_uo=0  BlockDataType=double  SampleTimeInherited=off  switch_inport=on
      settings: SourceProductName=MATLAB Runtime - Model Predictive Control Toolbox Addin  SourceProductBaseCode=Missing
  MPC2 : mpclib/MPC Controller  SCDEnableBlockLinearizationSpecification=on  mpcobj=fault1MPC  x0=[]  is_multiple=1  enable_value=2  return_u0=on  updateMPCinCallerWorkspace=on  md_inport=on  mv_inport=on  uref_inport=on  return_cost=on  return_mvseq=on  return_qpstatus=on  return_xseq=on  return_state=on  return_ovseq=on  state_inport=off  umin_inport=on  umax_inport=on  ymin_inport=on  ymax_inport=on  cc_inport=off  ywt_inport=on  uwt_inport=on  duwt_inport=on  rhoeps_inport=on  pm_inport=off  MaximumP=10  HorizonChoice=FixedHorizon  n_ts=0.05  n_p=10  n_mv=4  n_md=0  n_ud=0  n_mo=4  n_uo=0  BlockDataType=double  SampleTimeInherited=off  switch_inport=on
      settings: SourceProductName=MATLAB Runtime - Model Predictive Control Toolbox Addin  SourceProductBaseCode=Missing
  cost_switch : MultiPortSwitch  DiagnosticForDefault=None  SampleTime=mmpc_ts
  cost_terminator : Terminator
  cost_zero : Constant  Value=0  OutDataTypeStr=BlockDataType_multiple
  du.wt_zero : Constant  Value=zeros(4,1)  OutDataTypeStr=BlockDataType_multiple
  ecr.wt_zero : Constant  Value=zeros(1,1)  OutDataTypeStr=BlockDataType_multiple
  est.state_MPC2 : Terminator
  est.state_switch : MultiPortSwitch  DiagnosticForDefault=None  SampleTime=mmpc_ts
  est.state_terminator : Terminator
  est.state_zero : Constant  Value=mmpc_state  VectorParams1D=off  OutDataTypeStr=BlockDataType_multiple
  md_zero : Constant  Value=zeros(1,1)  OutDataTypeStr=BlockDataType_multiple
  mv.seq_MPC1 : Terminator
  mv.seq_MPC2 : Terminator
  mv.seq_switch : MultiPortSwitch  DiagnosticForDefault=None  SampleTime=mmpc_ts
  mv.seq_terminator : Terminator
  mv.seq_zero : Constant  Value=mmpc_mvseq  VectorParams1D=off  OutDataTypeStr=BlockDataType_multiple
  mv.target_zero : Constant  Value=zeros(4,1)  OutDataTypeStr=BlockDataType_multiple
  mv_switch : MultiPortSwitch  DiagnosticForDefault=None  SampleTime=mmpc_ts
  qp.status_switch : MultiPortSwitch  DiagnosticForDefault=None  SampleTime=mmpc_ts
  qp.status_terminator : Terminator
  qp.status_zero : Constant  Value=-1  OutDataTypeStr=BlockDataType_multiple
  u.wt_zero : Constant  Value=zeros(4,1)  OutDataTypeStr=BlockDataType_multiple
  u0_switch : MultiPortSwitch  DiagnosticForDefault=None  SampleTime=mmpc_ts
  u0_zero : Constant  Value=mmpc_u0  OutDataTypeStr=BlockDataType_multiple
  u[k-1] : Delay  DelayLength=1  InitialConditionSource=Input port
      settings: InputPortMap=u0,p4
  umax_zero : Constant  Value=zeros(4,1)  OutDataTypeStr=BlockDataType_multiple
  umin_zero : Constant  Value=zeros(4,1)  OutDataTypeStr=BlockDataType_multiple
  x.seq_MPC1 : Terminator
  x.seq_MPC2 : Terminator
  x.seq_switch : MultiPortSwitch  DiagnosticForDefault=None  SampleTime=mmpc_ts
  x.seq_terminator : Terminator
  x.seq_zero : Constant  Value=mmpc_xseq  VectorParams1D=off  OutDataTypeStr=BlockDataType_multiple
  y.seq_MPC1 : Terminator
  y.seq_MPC2 : Terminator
  y.seq_switch : MultiPortSwitch  DiagnosticForDefault=None  SampleTime=mmpc_ts
  y.seq_terminator : Terminator
  y.seq_zero : Constant  Value=mmpc_yseq  VectorParams1D=off  OutDataTypeStr=BlockDataType_multiple
  y.wt_zero : Constant  Value=zeros(4,1)  OutDataTypeStr=BlockDataType_multiple
  ymax_zero : Constant  Value=zeros(4,1)  OutDataTypeStr=BlockDataType_multiple
  ymin_zero : Constant  Value=zeros(4,1)  OutDataTypeStr=BlockDataType_multiple
  mv : Outport
  Out1 : Outport  Port=2
  wires:
  y.seq_zero/1 -> y.seq_switch/2, y.seq_switch/4, y.seq_switch/3
  x.seq_zero/1 -> x.seq_switch/4, x.seq_switch/3, x.seq_switch/2
  y.seq_switch/1 -> y.seq_terminator/1
  x.seq_switch/1 -> x.seq_terminator/1
  MPC1/6 -> qp.status_switch/2
  MPC1/5 -> y.seq_MPC1/1
  MPC1/4 -> x.seq_MPC1/1
  MPC1/3 -> mv.seq_MPC1/1
  MPC1/7 -> Out1/1
  est.state_zero/1 -> est.state_switch/2, est.state_switch/4, est.state_switch/3
  est.state_switch/1 -> est.state_terminator/1
  ecr.wt_zero/1 -> [M]
  du.wt_zero/1 -> [L]
  u.wt_zero/1 -> [K]
  y.wt_zero/1 -> [J]
  ymax_zero/1 -> [H]
  ymin_zero/1 -> [G]
  umax_zero/1 -> [F]
  umin_zero/1 -> [E]
  mv.target_zero/1 -> [N]
  u0_switch/1 -> u[k-1]/2
  u[k-1]/1 -> [D], mv_switch/4
  MPC1/8 -> u0_switch/2
  [M] -> MPC1/13, MPC2/13
  [I] -> MPC1/9, MPC2/9
  [J] -> MPC1/10, MPC2/10
  [L] -> MPC1/12, MPC2/12
  [K] -> MPC1/11, MPC2/11
  [H] -> MPC1/8, MPC2/8
  [G] -> MPC1/7, MPC2/7
  [F] -> MPC1/6, MPC2/6
  [E] -> MPC1/5, MPC2/5
  [N] -> MPC1/14, MPC2/14
  mv.seq_zero/1 -> mv.seq_switch/4, mv.seq_switch/3, mv.seq_switch/2
  qp.status_switch/1 -> qp.status_terminator/1
  mv.seq_switch/1 -> mv.seq_terminator/1
  MPC1/2 -> cost_switch/2
  cost_switch/1 -> cost_terminator/1
  [D] -> MPC1/4, MPC2/4
  [C] -> MPC1/3, MPC2/3
  [B] -> MPC1/2, MPC2/2
  [A] -> MPC1/1, MPC2/1
  switch/1 -> [I], cost_switch/1, mv.seq_switch/1, y.seq_switch/1, qp.status_switch/1, u0_switch/1, est.state_switch/1, x.seq_switch/1, mv_switch/1
  MPC1/1 -> mv_switch/2
  mv_switch/1 -> mv/1, u[k-1]/1
  mo or x/1 -> [A]
  ref/1 -> [B]
  md_zero/1 -> [C]
  cost_zero/1 -> cost_switch/4
  qp.status_zero/1 -> qp.status_switch/4
  u0_zero/1 -> u0_switch/4
  MPC2/1 -> mv_switch/3
  MPC2/2 -> cost_switch/3
  MPC2/3 -> mv.seq_MPC2/1
  MPC2/4 -> x.seq_MPC2/1
  MPC2/5 -> y.seq_MPC2/1
  MPC2/6 -> qp.status_switch/3
  MPC2/7 -> est.state_MPC2/1
  MPC2/8 -> u0_switch/3
